simulink model "Copy_of_compare"  (R2018b)
settings: Solver=ode45  StartTime=0.0  StopTime=100  RelTol=1e-3
libraries: neural x108
(part 2 of 4)

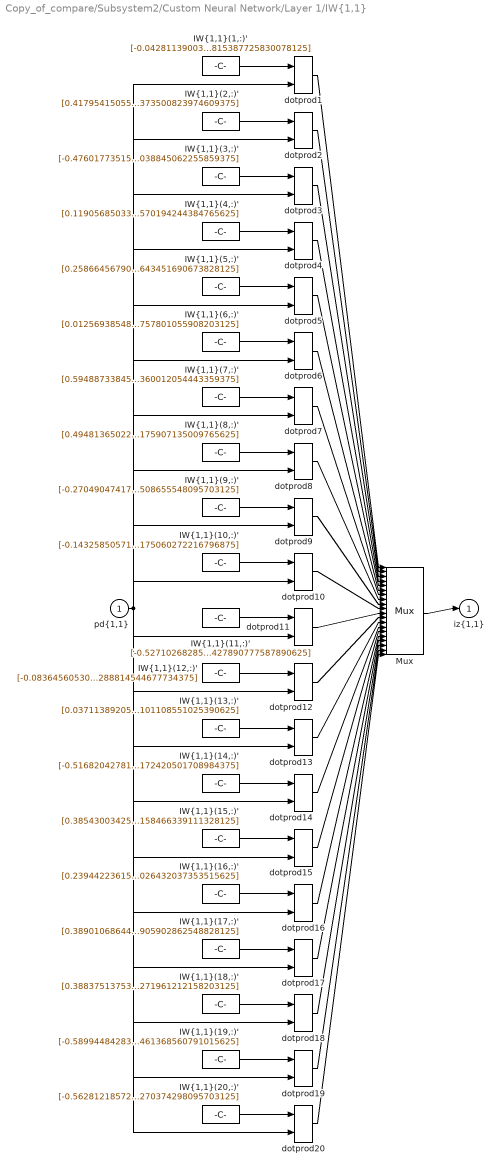
== system Copy_of_compare/Subsystem2/Custom Neural Network/Layer 1/IW{1,1} ==
  "pd{1,1}" : Inport  PortDimensions=4  SampleTime=1
      mask Display: e = 0.06;c1 = [120 230 180]/255;c2 = ([120 230 180]+0)/(256+128);c3 = ([120 230 180]+128)/(256+128);patch([0 1 1 0],[0 0 1 1],c1);patch([0 1 1 1-e 1-e 0+e],[0 0 1 1-e 0+e 0+e],c2);patch([0 0 1 1-e 0+e 0+e],[0 1 1 1-e 1-e 0+e],c3);plot([0 1 1 0 0],[0 0 1 1 0]);
  "IW{1,1}(1,:)'" : Constant  Value=[-0.042811390033023755119501174704055301845073699951171875;-0.34494124940580495053410459149745292961597442626953125;0.212181792987700124086813957546837627887725830078125;0.19703731840338456482442097694729454815387725830078125]
      mask Display: e = 0.06;c1 = [120 150 230]/255;c2 = ([120 150 230]+0)/383;c3 = ([120 150 230]+128)/383;patch([0 1 1 0],[0 0 1 1],c1);patch([0 1 1 1-e 1-e 0+e],[0 0 1 1-e 0+e 0+e],c2);patch([0 0 1 1-e 0+e 0+e],[0 1 1 1-e 1-e 0+e],c3);plot([0 1 1 0 0],[0 0 1 1 0]);disp('Weights');
  "IW{1,1}(10,:)'" : Constant  Value=[-0.1432585057147908458308194212804664857685565948486328125;-0.153266205858384185756193573979544453322887420654296875;0.49559029394590659034491864076699130237102508544921875;-0.07933482509106119795472267242075758986175060272216796875]
      mask Display: e = 0.06;c1 = [120 150 230]/255;c2 = ([120 150 230]+0)/383;c3 = ([120 150 230]+128)/383;patch([0 1 1 0],[0 0 1 1],c1);patch([0 1 1 1-e 1-e 0+e],[0 0 1 1-e 0+e 0+e],c2);patch([0 0 1 1-e 0+e 0+e],[0 1 1 1-e 1-e 0+e],c3);plot([0 1 1 0 0],[0 0 1 1 0]);disp('Weights');
  "IW{1,1}(11,:)'" : Constant  Value=[-0.5271026828588116774909622108680196106433868408203125;-0.19376380367271484050917251806822605431079864501953125;-0.50126266277864350850990149410790763795375823974609375;-0.1275131171211906500051469492973410524427890777587890625]
      mask Display: e = 0.06;c1 = [120 150 230]/255;c2 = ([120 150 230]+0)/383;c3 = ([120 150 230]+128)/383;patch([0 1 1 0],[0 0 1 1],c1);patch([0 1 1 1-e 1-e 0+e],[0 0 1 1-e 0+e 0+e],c2);patch([0 0 1 1-e 0+e 0+e],[0 1 1 1-e 1-e 0+e],c3);plot([0 1 1 0 0],[0 0 1 1 0]);disp('Weights');
  "IW{1,1}(12,:)'" : Constant  Value=[-0.083645605300920744529236117159598506987094879150390625;0.1272107414484172360769065335261984728276729583740234375;-0.1374343203091800968973501539949211291968822479248046875;0.66581955393483605032400873824371956288814544677734375]
      mask Display: e = 0.06;c1 = [120 150 230]/255;c2 = ([120 150 230]+0)/383;c3 = ([120 150 230]+128)/383;patch([0 1 1 0],[0 0 1 1],c1);patch([0 1 1 1-e 1-e 0+e],[0 0 1 1-e 0+e 0+e],c2);patch([0 0 1 1-e 0+e 0+e],[0 1 1 1-e 1-e 0+e],c3);plot([0 1 1 0 0],[0 0 1 1 0]);disp('Weights');
  "IW{1,1}(13,:)'" : Constant  Value=[0.03711389205480629394084957084487541578710079193115234375;-0.462899083442104508634429294033907353878021240234375;-0.2264716472284484527488501726111280731856822967529296875;0.4688615702267180385121037033968605101108551025390625]
      mask Display: e = 0.06;c1 = [120 150 230]/255;c2 = ([120 150 230]+0)/383;c3 = ([120 150 230]+128)/383;patch([0 1 1 0],[0 0 1 1],c1);patch([0 1 1 1-e 1-e 0+e],[0 0 1 1-e 0+e 0+e],c2);patch([0 0 1 1-e 0+e 0+e],[0 1 1 1-e 1-e 0+e],c3);plot([0 1 1 0 0],[0 0 1 1 0]);disp('Weights');
  "IW{1,1}(14,:)'" : Constant  Value=[-0.5168204278140742236047344704275019466876983642578125;0.45663111946031242904808777893777005374431610107421875;-0.51419835913847655728403651664848439395427703857421875;-0.09691171847871636602089751022504060529172420501708984375]
      mask Display: e = 0.06;c1 = [120 150 230]/255;c2 = ([120 150 230]+0)/383;c3 = ([120 150 230]+128)/383;patch([0 1 1 0],[0 0 1 1],c1);patch([0 1 1 1-e 1-e 0+e],[0 0 1 1-e 0+e 0+e],c2);patch([0 0 1 1-e 0+e 0+e],[0 1 1 1-e 1-e 0+e],c3);plot([0 1 1 0 0],[0 0 1 1 0]);disp('Weights');
  "IW{1,1}(15,:)'" : Constant  Value=[0.385430034255971387668893157751881517469882965087890625;-0.215305325209396214436452510199160315096378326416015625;-0.1868848258074100876502399160017375834286212921142578125;0.39665474045523041457528279352118261158466339111328125]
      mask Display: e = 0.06;c1 = [120 150 230]/255;c2 = ([120 150 230]+0)/383;c3 = ([120 150 230]+128)/383;patch([0 1 1 0],[0 0 1 1],c1);patch([0 1 1 1-e 1-e 0+e],[0 0 1 1-e 0+e 0+e],c2);patch([0 0 1 1-e 0+e 0+e],[0 1 1 1-e 1-e 0+e],c3);plot([0 1 1 0 0],[0 0 1 1 0]);disp('Weights');
  "IW{1,1}(16,:)'" : Constant  Value=[0.2394422361532615173285165610650437884032726287841796875;0.5573707637317522056719099055044353008270263671875;-0.44328627858535185612964824031223542988300323486328125;-0.20052230029704232183718204396427609026432037353515625]
      mask Display: e = 0.06;c1 = [120 150 230]/255;c2 = ([120 150 230]+0)/383;c3 = ([120 150 230]+128)/383;patch([0 1 1 0],[0 0 1 1],c1);patch([0 1 1 1-e 1-e 0+e],[0 0 1 1-e 0+e 0+e],c2);patch([0 0 1 1-e 0+e 0+e],[0 1 1 1-e 1-e 0+e],c3);plot([0 1 1 0 0],[0 0 1 1 0]);disp('Weights');
  "IW{1,1}(17,:)'" : Constant  Value=[0.38901068644869807311437170938006602227687835693359375;-0.427525166182410376602973656190442852675914764404296875;-0.443132878250084905058514550546533428132534027099609375;0.37252488448668785725459429158945567905902862548828125]
      mask Display: e = 0.06;c1 = [120 150 230]/255;c2 = ([120 150 230]+0)/383;c3 = ([120 150 230]+128)/383;patch([0 1 1 0],[0 0 1 1],c1);patch([0 1 1 1-e 1-e 0+e],[0 0 1 1-e 0+e 0+e],c2);patch([0 0 1 1-e 0+e 0+e],[0 1 1 1-e 1-e 0+e],c3);plot([0 1 1 0 0],[0 0 1 1 0]);disp('Weights');
  "IW{1,1}(18,:)'" : Constant  Value=[0.38837513753777053171489797023241408169269561767578125;-0.329414929396628364255406040683737955987453460693359375;0.447224063257221360334625614996184594929218292236328125;-0.293902664542561364857675698658567853271961212158203125]
      mask Display: e = 0.06;c1 = [120 150 230]/255;c2 = ([120 150 230]+0)/383;c3 = ([120 150 230]+128)/383;patch([0 1 1 0],[0 0 1 1],c1);patch([0 1 1 1-e 1-e 0+e],[0 0 1 1-e 0+e 0+e],c2);patch([0 0 1 1-e 0+e 0+e],[0 1 1 1-e 1-e 0+e],c3);plot([0 1 1 0 0],[0 0 1 1 0]);disp('Weights');
  "IW{1,1}(19,:)'" : Constant  Value=[-0.58994484283590320483625646375003270804882049560546875;-0.4543619457979339859576839444343931972980499267578125;-0.38699246687251276366481533841579221189022064208984375;-0.1299714765164118601692422316773445345461368560791015625]
      mask Display: e = 0.06;c1 = [120 150 230]/255;c2 = ([120 150 230]+0)/383;c3 = ([120 150 230]+128)/383;patch([0 1 1 0],[0 0 1 1],c1);patch([0 1 1 1-e 1-e 0+e],[0 0 1 1-e 0+e 0+e],c2);patch([0 0 1 1-e 0+e 0+e],[0 1 1 1-e 1-e 0+e],c3);plot([0 1 1 0 0],[0 0 1 1 0]);disp('Weights');
  "IW{1,1}(2,:)'" : Constant  Value=[0.417954150552907910398658941630856133997440338134765625;0.37950717584964566153615805887966416776180267333984375;-0.444355699691141747820211094222031533718109130859375;0.40455774770315766630801590508781373500823974609375]
      mask Display: e = 0.06;c1 = [120 150 230]/255;c2 = ([120 150 230]+0)/383;c3 = ([120 150 230]+128)/383;patch([0 1 1 0],[0 0 1 1],c1);patch([0 1 1 1-e 1-e 0+e],[0 0 1 1-e 0+e 0+e],c2);patch([0 0 1 1-e 0+e 0+e],[0 1 1 1-e 1-e 0+e],c3);plot([0 1 1 0 0],[0 0 1 1 0]);disp('Weights');
  "IW{1,1}(20,:)'" : Constant  Value=[-0.56281218572056845861339979819604195654392242431640625;-0.1531865678348197923330786807127879001200199127197265625;0.32894636374948527102191064841463230550289154052734375;-0.11506127596662703294061458336727810092270374298095703125]
      mask Display: e = 0.06;c1 = [120 150 230]/255;c2 = ([120 150 230]+0)/383;c3 = ([120 150 230]+128)/383;patch([0 1 1 0],[0 0 1 1],c1);patch([0 1 1 1-e 1-e 0+e],[0 0 1 1-e 0+e 0+e],c2);patch([0 0 1 1-e 0+e 0+e],[0 1 1 1-e 1-e 0+e],c3);plot([0 1 1 0 0],[0 0 1 1 0]);disp('Weights');
  "IW{1,1}(3,:)'" : Constant  Value=[-0.476017735150680909583797983941622078418731689453125;0.372659870345571853089694513982976786792278289794921875;0.15761264234491967339835127859259955585002899169921875;-0.301498932852593437559107769629918038845062255859375]
      mask Display: e = 0.06;c1 = [120 150 230]/255;c2 = ([120 150 230]+0)/383;c3 = ([120 150 230]+128)/383;patch([0 1 1 0],[0 0 1 1],c1);patch([0 1 1 1-e 1-e 0+e],[0 0 1 1-e 0+e 0+e],c2);patch([0 0 1 1-e 0+e 0+e],[0 1 1 1-e 1-e 0+e],c3);plot([0 1 1 0 0],[0 0 1 1 0]);disp('Weights');
  "IW{1,1}(4,:)'" : Constant  Value=[0.1190568503323596039056297968272701837122440338134765625;0.025251810519317963166230356364394538104534149169921875;-0.01463313633015732827258315040808156481944024562835693359375;0.0799177967721290960501079325695172883570194244384765625]
      mask Display: e = 0.06;c1 = [120 150 230]/255;c2 = ([120 150 230]+0)/383;c3 = ([120 150 230]+128)/383;patch([0 1 1 0],[0 0 1 1],c1);patch([0 1 1 1-e 1-e 0+e],[0 0 1 1-e 0+e 0+e],c2);patch([0 0 1 1-e 0+e 0+e],[0 1 1 1-e 1-e 0+e],c3);plot([0 1 1 0 0],[0 0 1 1 0]);disp('Weights');
  "IW{1,1}(5,:)'" : Constant  Value=[0.2586645679057075764006867757416330277919769287109375;-0.359798037926290892318803571470198221504688262939453125;0.49791321437721602904957762802951037883758544921875;-0.2408924072199911947667061440370162017643451690673828125]
      mask Display: e = 0.06;c1 = [120 150 230]/255;c2 = ([120 150 230]+0)/383;c3 = ([120 150 230]+128)/383;patch([0 1 1 0],[0 0 1 1],c1);patch([0 1 1 1-e 1-e 0+e],[0 0 1 1-e 0+e 0+e],c2);patch([0 0 1 1-e 0+e 0+e],[0 1 1 1-e 1-e 0+e],c3);plot([0 1 1 0 0],[0 0 1 1 0]);disp('Weights');
  "IW{1,1}(6,:)'" : Constant  Value=[0.01256938548635226811367449073486568522639572620391845703125;0.422855987628569407466017082697362639009952545166015625;0.482605939133784911376778836711309850215911865234375;-0.478909325852367839804202276354772038757801055908203125]
      mask Display: e = 0.06;c1 = [120 150 230]/255;c2 = ([120 150 230]+0)/383;c3 = ([120 150 230]+128)/383;patch([0 1 1 0],[0 0 1 1],c1);patch([0 1 1 1-e 1-e 0+e],[0 0 1 1-e 0+e 0+e],c2);patch([0 0 1 1-e 0+e 0+e],[0 1 1 1-e 1-e 0+e],c3);plot([0 1 1 0 0],[0 0 1 1 0]);disp('Weights');
  "IW{1,1}(7,:)'" : Constant  Value=[0.5948873384524977492304742554551921784877777099609375;0.281306962804711513381761278651538304984569549560546875;-0.1572109737119190830956227955539361573755741119384765625;0.1660798915358044636203516120076528750360012054443359375]
      mask Display: e = 0.06;c1 = [120 150 230]/255;c2 = ([120 150 230]+0)/383;c3 = ([120 150 230]+128)/383;patch([0 1 1 0],[0 0 1 1],c1);patch([0 1 1 1-e 1-e 0+e],[0 0 1 1-e 0+e 0+e],c2);patch([0 0 1 1-e 0+e 0+e],[0 1 1 1-e 1-e 0+e],c3);plot([0 1 1 0 0],[0 0 1 1 0]);disp('Weights');
  "IW{1,1}(8,:)'" : Constant  Value=[0.494813650227310108942191391179221682250499725341796875;-0.1661270735577930202087060251869843341410160064697265625;-0.323120860559985623172707391859148629009723663330078125;-0.120857806854206606406165747102932073175907135009765625]
      mask Display: e = 0.06;c1 = [120 150 230]/255;c2 = ([120 150 230]+0)/383;c3 = ([120 150 230]+128)/383;patch([0 1 1 0],[0 0 1 1],c1);patch([0 1 1 1-e 1-e 0+e],[0 0 1 1-e 0+e 0+e],c2);patch([0 0 1 1-e 0+e 0+e],[0 1 1 1-e 1-e 0+e],c3);plot([0 1 1 0 0],[0 0 1 1 0]);disp('Weights');
  "IW{1,1}(9,:)'" : Constant  Value=[-0.27049047417204652443700751973665319383144378662109375;-0.030493674231205934732624740490791737101972103118896484375;-0.30275890613240985516085856943391263484954833984375;0.32392632672577914565437140481662936508655548095703125]
      mask Display: e = 0.06;c1 = [120 150 230]/255;c2 = ([120 150 230]+0)/383;c3 = ([120 150 230]+128)/383;patch([0 1 1 0],[0 0 1 1],c1);patch([0 1 1 1-e 1-e 0+e],[0 0 1 1-e 0+e 0+e],c2);patch([0 0 1 1-e 0+e 0+e],[0 1 1 1-e 1-e 0+e],c3);plot([0 1 1 0 0],[0 0 1 1 0]);disp('Weights');
  Mux : Mux  Inputs=20
      mask Display: e = 0.06;c1 = [120 150 230]/255;c2 = ([120 150 230]+0)/383;c3 = ([120 150 230]+128)/383;patch([0 1 1 0],[0 0 1 1],c1);patch([0 1 1 1-e 1-e 0+e],[0 0 1 1-e 0+e 0+e],c2);patch([0 0 1 1-e 0+e 0+e],[0 1 1 1-e 1-e 0+e],c3);plot([0 1 1 0 0],[0 0 1 1 0]);disp('Mux');
  dotprod{1..20} (20 alike) : neural/Weight Functions/dotprod
  "iz{1,1}" : Outport
      mask Display: e = 0.06;c1 = [120 230 180]/255;c2 = ([120 230 180]+0)/(256+128);c3 = ([120 230 180]+128)/(256+128);patch([0 1 1 0],[0 0 1 1],c1);patch([0 1 1 1-e 1-e 0+e],[0 0 1 1-e 0+e 0+e],c2);patch([0 0 1 1-e 0+e 0+e],[0 1 1 1-e 1-e 0+e],c3);plot([0 1 1 0 0],[0 0 1 1 0]);
  wires:
  "IW{1,1}(1,:)'"/1 -> dotprod1/1
  "pd{1,1}"/1 -> dotprod1/2, dotprod2/2, dotprod3/2, dotprod4/2, dotprod5/2, dotprod6/2, dotprod7/2, dotprod8/2, dotprod9/2, dotprod10/2, dotprod11/2, dotprod12/2, dotprod13/2, dotprod14/2, dotprod15/2, dotprod16/2, dotprod17/2, dotprod18/2, dotprod19/2, dotprod20/2
  dotprod1/1 -> Mux/1
  "IW{1,1}(2,:)'"/1 -> dotprod2/1
  dotprod2/1 -> Mux/2
  "IW{1,1}(3,:)'"/1 -> dotprod3/1
  dotprod3/1 -> Mux/3
  "IW{1,1}(4,:)'"/1 -> dotprod4/1
  dotprod4/1 -> Mux/4
  "IW{1,1}(5,:)'"/1 -> dotprod5/1
  dotprod5/1 -> Mux/5
  "IW{1,1}(6,:)'"/1 -> dotprod6/1
  dotprod6/1 -> Mux/6
  "IW{1,1}(7,:)'"/1 -> dotprod7/1
  dotprod7/1 -> Mux/7
  "IW{1,1}(8,:)'"/1 -> dotprod8/1
  dotprod8/1 -> Mux/8
  "IW{1,1}(9,:)'"/1 -> dotprod9/1
  dotprod9/1 -> Mux/9
  "IW{1,1}(10,:)'"/1 -> dotprod10/1
  dotprod10/1 -> Mux/10
  "IW{1,1}(11,:)'"/1 -> dotprod11/1
  dotprod11/1 -> Mux/11
  "IW{1,1}(12,:)'"/1 -> dotprod12/1
  dotprod12/1 -> Mux/12
  "IW{1,1}(13,:)'"/1 -> dotprod13/1
  dotprod13/1 -> Mux/13
  "IW{1,1}(14,:)'"/1 -> dotprod14/1
  dotprod14/1 -> Mux/14
  "IW{1,1}(15,:)'"/1 -> dotprod15/1
  dotprod15/1 -> Mux/15
  "IW{1,1}(16,:)'"/1 -> dotprod16/1
  dotprod16/1 -> Mux/16
  "IW{1,1}(17,:)'"/1 -> dotprod17/1
  dotprod17/1 -> Mux/17
  "IW{1,1}(18,:)'"/1 -> dotprod18/1
  dotprod18/1 -> Mux/18
  "IW{1,1}(19,:)'"/1 -> dotprod19/1
  dotprod19/1 -> Mux/19
  "IW{1,1}(20,:)'"/1 -> dotprod20/1
  dotprod20/1 -> Mux/20
  Mux/1 -> "iz{1,1}"/1

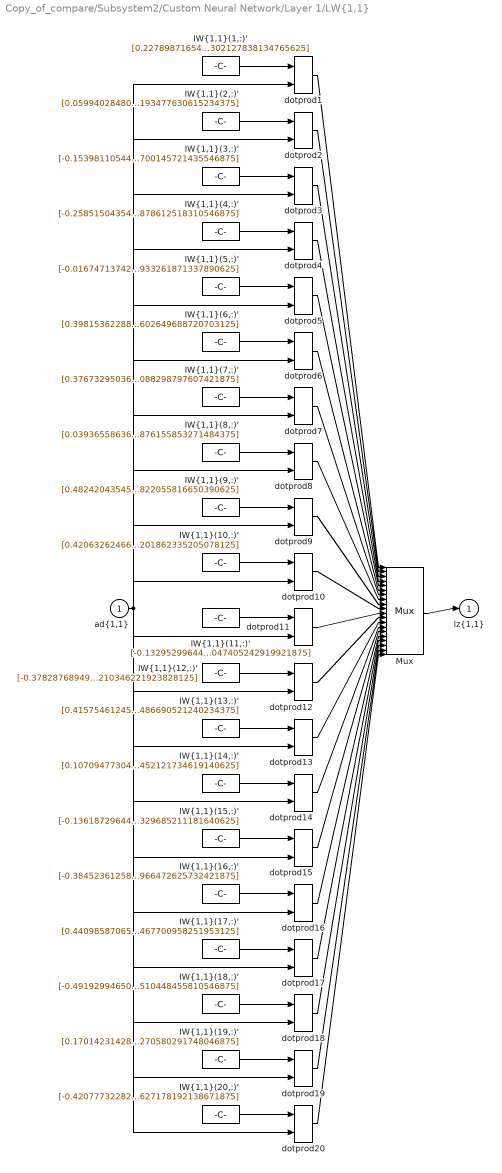
== system Copy_of_compare/Subsystem2/Custom Neural Network/Layer 1/LW{1,1} ==
  "ad{1,1}" : Inport  PortDimensions=20  SampleTime=1
      mask Display: e = 0.06;c1 = [120 230 180]/255;c2 = ([120 230 180]+0)/(256+128);c3 = ([120 230 180]+128)/(256+128);patch([0 1 1 0],[0 0 1 1],c1);patch([0 1 1 1-e 1-e 0+e],[0 0 1 1-e 0+e 0+e],c2);patch([0 0 1 1-e 0+e 0+e],[0 1 1 1-e 1-e 0+e],c3);plot([0 1 1 0 0],[0 0 1 1 0]);
  "IW{1,1}(1,:)'" : Constant  Value=[0.2278987165494096578388649732005433179438114166259765625;0.240540154904058389728760403158958069980144500732421875;-0.08228071789715719897007062400007271207869052886962890625;0.4457988335202587304451071759103797376155853271484375;-0.23129699864569508438449929599300958216190338134765625;-0.49692828504273933720725153762032277882099151611328125;0.38560473208843759618247304388205520808696746826171875;0.31956777070472852653182371795992366969585418701171875;0.1656064949527651652960713590800878591835498809814453125;0.229070693094035660042351310039521194994449615478515625;-0.475851979993766105447861036736867390573024749755859375;0.31630195271679417690080526881502009928226470947265625;0.49015943893010571752455462046782486140727996826171875;-0.50065157873258236964630896181915886700153350830078125;-0.45776780495111413227249386181938461959362030029296875;0.2098533389682639693774035549722611904144287109375;0.38657180100997201588342022660071961581707000732421875;0.240641344614608454488546840366325341165065765380859375;-0.30911232252311748869288976493407972157001495361328125;0.07903324281619496238793232123498455621302127838134765625]
      mask Display: e = 0.06;c1 = [120 150 230]/255;c2 = ([120 150 230]+0)/383;c3 = ([120 150 230]+128)/383;patch([0 1 1 0],[0 0 1 1],c1);patch([0 1 1 1-e 1-e 0+e],[0 0 1 1-e 0+e 0+e],c2);patch([0 0 1 1-e 0+e 0+e],[0 1 1 1-e 1-e 0+e],c3);plot([0 1 1 0 0],[0 0 1 1 0]);disp('weights');
  "IW{1,1}(10,:)'" : Constant  Value=[0.420632624664030119188140588448732160031795501708984375;0.429185444508361990667566487900330685079097747802734375;-0.491659080709817175591780369359184987843036651611328125;0.182452654614607079341936923810862936079502105712890625;-0.10699046596342180748262506995160947553813457489013671875;0.1602960437006126503955982798288459889590740203857421875;-0.38946695359310312678502441485761664807796478271484375;-0.23785342454607505402464084909297525882720947265625;0.09697167013946524083412015215799328871071338653564453125;-0.2307044267848055996150691271395771764218807220458984375;0.27990512871394057636820207335404120385646820068359375;0.3074695770440818431978868829901330173015594482421875;-0.49869450365044720729912341994349844753742218017578125;0.212638380584271258211259691961458884179592132568359375;0.0196244391094952570775422628912565414793789386749267578125;-0.155944109151455012618470163943129591643810272216796875;0.469563664574393968553778222485561855137348175048828125;0.271650147852854517704912495901226066052913665771484375;0.514697400127334336872308995225466787815093994140625;-0.463282954366107724286649727218900807201862335205078125]
      mask Display: e = 0.06;c1 = [120 150 230]/255;c2 = ([120 150 230]+0)/383;c3 = ([120 150 230]+128)/383;patch([0 1 1 0],[0 0 1 1],c1);patch([0 1 1 1-e 1-e 0+e],[0 0 1 1-e 0+e 0+e],c2);patch([0 0 1 1-e 0+e 0+e],[0 1 1 1-e 1-e 0+e],c3);plot([0 1 1 0 0],[0 0 1 1 0]);disp('weights');
  "IW{1,1}(11,:)'" : Constant  Value=[-0.13295299644515246040299416563357226550579071044921875;-0.34257970274611437844214378856122493743896484375;-0.50546742207309069971898907169816084206104278564453125;0.375317987307353051473768346113502047955989837646484375;0.293111656529973618745543717523105442523956298828125;-0.4780711225226854654835051405825652182102203369140625;-0.29780200740318452101718094127136282622814178466796875;0.12431875943552746222042770796178956516087055206298828125;0.1488731855108570700796377650476642884314060211181640625;0.47588212639451510366228603743365965783596038818359375;-0.2544601172016609513804041853290982544422149658203125;-0.387733186112341365880951116196229122579097747802734375;-0.178865737611743902402139383411849848926067352294921875;-0.36554438569003178116645358386449515819549560546875;0.265494376935527187644225932672270573675632476806640625;-0.145739478578150116749867493126657791435718536376953125;-0.1630710952019509552002318741870112717151641845703125;-0.420982141038813761912962263522786088287830352783203125;-0.318278423537587451530583848580135963857173919677734375;-0.08046330758533119797970556419386412017047405242919921875]
      mask Display: e = 0.06;c1 = [120 150 230]/255;c2 = ([120 150 230]+0)/383;c3 = ([120 150 230]+128)/383;patch([0 1 1 0],[0 0 1 1],c1);patch([0 1 1 1-e 1-e 0+e],[0 0 1 1-e 0+e 0+e],c2);patch([0 0 1 1-e 0+e 0+e],[0 1 1 1-e 1-e 0+e],c3);plot([0 1 1 0 0],[0 0 1 1 0]);disp('weights');
  "IW{1,1}(12,:)'" : Constant  Value=[-0.378287689491962009213921191985718905925750732421875;0.31412463184470540422665862934081815183162689208984375;-0.245211026062742920572645743959583342075347900390625;-0.347387547677588059968911693431437015533447265625;-0.5031677654191166748631758309784345328807830810546875;-0.50758261729631259928652298185625113546848297119140625;0.37116161778317968700235951473587192595005035400390625;-0.03775716422149082152071031259765732102096080780029296875;-0.04605910262436473112668267049230053089559078216552734375;0.0104202638426654503600587986511527560651302337646484375;0.1388820306765665979487067716036108322441577911376953125;0.32356457862817589177240051867556758224964141845703125;0.00903262123542868111680803622220992110669612884521484375;0.545086378847996488872240661294199526309967041015625;0.054844572033606098226954372876207344233989715576171875;-0.12227603828467183133543727535652578808367252349853515625;0.52393929318664655969683963121497072279453277587890625;-0.1110905758660236941626209272726555354893207550048828125;0.54684918251084091433966705153579823672771453857421875;-0.241502604628337724790299034793861210346221923828125]
      mask Display: e = 0.06;c1 = [120 150 230]/255;c2 = ([120 150 230]+0)/383;c3 = ([120 150 230]+128)/383;patch([0 1 1 0],[0 0 1 1],c1);patch([0 1 1 1-e 1-e 0+e],[0 0 1 1-e 0+e 0+e],c2);patch([0 0 1 1-e 0+e 0+e],[0 1 1 1-e 1-e 0+e],c3);plot([0 1 1 0 0],[0 0 1 1 0]);disp('weights');
  "IW{1,1}(13,:)'" : Constant  Value=[0.41575461245577349789215304554090835154056549072265625;-0.409758839927184037588148157738032750785350799560546875;0.0292141310860018731110354650581939495168626308441162109375;0.32632919895820433620059475288144312798976898193359375;-0.39978185631407348044064065106795169413089752197265625;-0.419945798962307659252246594405733048915863037109375;-0.1446788768866233698684453656824189238250255584716796875;-0.33483109447959369386893513365066610276699066162109375;-0.039567165528868041002308331144377007149159908294677734375;0.29233486785391515905274673059466294944286346435546875;-0.322702359571785724057235711370594799518585205078125;0.346982308737791067532185707023018039762973785400390625;-0.00956612543968184993181669284467716352082788944244384765625;-0.3877596423322573482295183566748164594173431396484375;-0.35300446726813017317425646979245357215404510498046875;0.2962997531462061573392929858528077602386474609375;-0.40146500486877789715123299174592830240726470947265625;-0.377307450578544034680561480854521505534648895263671875;0.407805095951260521136561010280274786055088043212890625;-0.1819632532644864519877359043675824068486690521240234375]
      mask Display: e = 0.06;c1 = [120 150 230]/255;c2 = ([120 150 230]+0)/383;c3 = ([120 150 230]+128)/383;patch([0 1 1 0],[0 0 1 1],c1);patch([0 1 1 1-e 1-e 0+e],[0 0 1 1-e 0+e 0+e],c2);patch([0 0 1 1-e 0+e 0+e],[0 1 1 1-e 1-e 0+e],c3);plot([0 1 1 0 0],[0 0 1 1 0]);disp('weights');
  "IW{1,1}(14,:)'" : Constant  Value=[0.1070947730439226475152025841452996246516704559326171875;-0.271684022564260552190518183124368079006671905517578125;0.28236026004421599377991469737025909125804901123046875;0.2240856228544926553869487406700500287115573883056640625;-0.424180068223444506347874494167626835405826568603515625;0.09805112035332404218923585403899778611958026885986328125;-0.257571951610501781448903102500480599701404571533203125;-0.0929025916780819860374407426206744275987148284912109375;0.463081155692898149833780507833580486476421356201171875;0.32611395715227597946750393020920455455780029296875;-0.27906063380379120264507264437270350754261016845703125;-0.461085781794401849964515349711291491985321044921875;0.077706195310071723980627211858518421649932861328125;-0.30058122236647388803021385683678090572357177734375;0.4548280591144233664380180925945751368999481201171875;0.1008924803782029477883241952440585009753704071044921875;-0.375142648760853791856106909108348190784454345703125;-0.41173315079330163879234305568388663232326507568359375;-0.262394554640659916078249125348520465195178985595703125;-0.056615575605880132104008595206323661841452121734619140625]
      mask Display: e = 0.06;c1 = [120 150 230]/255;c2 = ([120 150 230]+0)/383;c3 = ([120 150 230]+128)/383;patch([0 1 1 0],[0 0 1 1],c1);patch([0 1 1 1-e 1-e 0+e],[0 0 1 1-e 0+e 0+e],c2);patch([0 0 1 1-e 0+e 0+e],[0 1 1 1-e 1-e 0+e],c3);plot([0 1 1 0 0],[0 0 1 1 0]);disp('weights');
  "IW{1,1}(15,:)'" : Constant  Value=[-0.136187296441313610007028955806163139641284942626953125;0.209037331339636534011106050456874072551727294921875;-0.32626772882534027520051722603966481983661651611328125;-0.462079150500124213873931466878275386989116668701171875;-0.285236058869271780213949796234373934566974639892578125;0.1559960849596407073125448050632257945835590362548828125;0.36825294505482997209355744416825473308563232421875;0.18261079235679178456308591194101609289646148681640625;0.0492753080605025928218054787066648714244365692138671875;0.138081756097673480354615094256587326526641845703125;0.07186485845076993894675609908517799340188503265380859375;-0.4007107673316190332712949384585954248905181884765625;0.430359673196610781342741347543778829276561737060546875;0.4609101603710115124812318754266016185283660888671875;-0.404191060521045975040266284850076772272586822509765625;-0.334065431476544050237720284712850116193294525146484375;-0.447605082750429150717508264278876595199108123779296875;-0.424280447044566688674649412860162556171417236328125;-0.372089526528038394559416701667942106723785400390625;-0.1983326147027272556844224027372547425329685211181640625]
      mask Display: e = 0.06;c1 = [120 150 230]/255;c2 = ([120 150 230]+0)/383;c3 = ([120 150 230]+128)/383;patch([0 1 1 0],[0 0 1 1],c1);patch([0 1 1 1-e 1-e 0+e],[0 0 1 1-e 0+e 0+e],c2);patch([0 0 1 1-e 0+e 0+e],[0 1 1 1-e 1-e 0+e],c3);plot([0 1 1 0 0],[0 0 1 1 0]);disp('weights');
  "IW{1,1}(16,:)'" : Constant  Value=[-0.384523612583706597689570116926915943622589111328125;-0.206157590542222102225622393234516493976116180419921875;0.4554611951382001588939374414621852338314056396484375;0.49174573636799523423945856848149560391902923583984375;-0.1801231476021115385233173356027691625058650970458984375;0.4683739136963203097963059917674399912357330322265625;0.394822850463422636568822099434328265488147735595703125;0.391845140376515799207624013433814980089664459228515625;0.06459290894014728390271073976691695861518383026123046875;-0.34207481769281422590012198270414955914020538330078125;-0.490312179861580654804953383063548244535923004150390625;-0.045903438096631769826938551659623044542968273162841796875;0.439061671021340360621110221472918055951595306396484375;0.10461216405642752291793584618062595836818218231201171875;0.2258046443601937625089703942649066448211669921875;-0.416842953303650565199944821870303712785243988037109375;0.18497573731176597533476524404250085353851318359375;0.06843741391665482398654063445064821280539035797119140625;-0.108158723682227952966883322005742229521274566650390625;0.19655617248948764608229566874797455966472625732421875]
      mask Display: e = 0.06;c1 = [120 150 230]/255;c2 = ([120 150 230]+0)/383;c3 = ([120 150 230]+128)/383;patch([0 1 1 0],[0 0 1 1],c1);patch([0 1 1 1-e 1-e 0+e],[0 0 1 1-e 0+e 0+e],c2);patch([0 0 1 1-e 0+e 0+e],[0 1 1 1-e 1-e 0+e],c3);plot([0 1 1 0 0],[0 0 1 1 0]);disp('weights');
  "IW{1,1}(17,:)'" : Constant  Value=[0.44098587065739192070168428472243249416351318359375;-0.08788059273859938347328579766326583921909332275390625;-0.308675876398948501044827708028606139123439788818359375;-0.221486569567091506893774521813611499965190887451171875;0.2178678865951073628792755698668770492076873779296875;-0.289200773370994423938640238702646456658840179443359375;0.35306632808482019125762008115998469293117523193359375;-0.444884415917694620024036566974245943129062652587890625;-0.199324943462346693134890074361464940011501312255859375;-0.08840657649147143359869005507789552211761474609375;-0.4380941991671647439687831138144247233867645263671875;0.01346592043859511089731739730268600396811962127685546875;-0.47008827633134420143079523768392391502857208251953125;-0.20000214664542592668539100486668758094310760498046875;0.2742024362016126648455838221707381308078765869140625;-0.37841706486119919272681499933241866528987884521484375;0.01755574999820135040362600875596399419009685516357421875;-0.335116990061384678600830966388457454741001129150390625;0.16408210758615771052149057140923105180263519287109375;0.44147467938079476557078351106611080467700958251953125]
      mask Display: e = 0.06;c1 = [120 150 230]/255;c2 = ([120 150 230]+0)/383;c3 = ([120 150 230]+128)/383;patch([0 1 1 0],[0 0 1 1],c1);patch([0 1 1 1-e 1-e 0+e],[0 0 1 1-e 0+e 0+e],c2);patch([0 0 1 1-e 0+e 0+e],[0 1 1 1-e 1-e 0+e],c3);plot([0 1 1 0 0],[0 0 1 1 0]);disp('weights');
  "IW{1,1}(18,:)'" : Constant  Value=[-0.491929946506200088673921300141955725848674774169921875;-0.2126767242213216391188979059734265320003032684326171875;-0.1009912537251317077302559255258529447019100189208984375;0.3217560834001089720146637773723341524600982666015625;0.051956008299841281716791030476088053546845912933349609375;-0.1660321893331526965642552795543451793491840362548828125;0.0272606663276684334229482686851042672060430049896240234375;0.491487382911402981289228364403243176639080047607421875;-0.354138503368337353993666738460888154804706573486328125;0.2047296393810319747874615359251038171350955963134765625;0.423050942762800030738645773453754372894763946533203125;0.370056287706793940461835745736607350409030914306640625;0.04510904995247948245928881760846707038581371307373046875;-0.403977073562105160053903318839729763567447662353515625;0.238067026591629649079351338514243252575397491455078125;0.460926551166004505599715912467218004167079925537109375;0.307803449094200265445664399521774612367153167724609375;-0.444383412258365917413271972691291011869907379150390625;-0.1183301293074575932795511334916227497160434722900390625;0.223305523038261621859845718063297681510448455810546875]
      mask Display: e = 0.06;c1 = [120 150 230]/255;c2 = ([120 150 230]+0)/383;c3 = ([120 150 230]+128)/383;patch([0 1 1 0],[0 0 1 1],c1);patch([0 1 1 1-e 1-e 0+e],[0 0 1 1-e 0+e 0+e],c2);patch([0 0 1 1-e 0+e 0+e],[0 1 1 1-e 1-e 0+e],c3);plot([0 1 1 0 0],[0 0 1 1 0]);disp('weights');
  "IW{1,1}(19,:)'" : Constant  Value=[0.1701423142892309059437394580527325160801410675048828125;-0.411160005228003611055243027294636704027652740478515625;0.04775542972130684959974900039014755748212337493896484375;0.2284830513994409451061784466219251044094562530517578125;-0.07416597601648027004994645494662108831107616424560546875;0.058993659299435431686564612618894898332655429840087890625;-0.043994833927363745373906311897371779195964336395263671875;0.5347552742001904224622421679669059813022613525390625;-0.205233087407502790000535242143087089061737060546875;-0.06123054241270009523390172034851275384426116943359375;0.2382264629099061503669787498438381589949131011962890625;-0.2471133906297690863151927942453767172992229461669921875;-0.354185081063232154452435906932805664837360382080078125;-0.56028937632563480253367060868185944855213165283203125;0.242926896839649353321277658324106596410274505615234375;-0.202115344162328958166341408286825753748416900634765625;0.55654225518627431501528235457953996956348419189453125;-0.1141277041438499839642872757394798099994659423828125;0.298276236068890365782380058590206317603588104248046875;-0.42325436819033679380908097300562076270580291748046875]
      mask Display: e = 0.06;c1 = [120 150 230]/255;c2 = ([120 150 230]+0)/383;c3 = ([120 150 230]+128)/383;patch([0 1 1 0],[0 0 1 1],c1);patch([0 1 1 1-e 1-e 0+e],[0 0 1 1-e 0+e 0+e],c2);patch([0 0 1 1-e 0+e 0+e],[0 1 1 1-e 1-e 0+e],c3);plot([0 1 1 0 0],[0 0 1 1 0]);disp('weights');
  "IW{1,1}(2,:)'" : Constant  Value=[0.05994028480322521890144571443670429289340972900390625;-0.08139306170899605896718043140936060808598995208740234375;0.37859367841592528325378452791483141481876373291015625;-0.28921655327229156551283040244015865027904510498046875;-0.392439976848181715229912924769450910389423370361328125;0.396248727965390068472828488665982149541378021240234375;-0.3554873052677731681825434861821122467517852783203125;-0.2112195004145205612378077830726397223770618438720703125;0.08326096933293403168363511213101446628570556640625;0.37248571015998155342430209202575497329235076904296875;0.43360619759672258677341005750349722802639007568359375;0.282109436908400679211439410210005007684230804443359375;0.3373217412508566770412699042935855686664581298828125;0.1598161592246870321698537509291782043874263763427734375;0.451645495361196636086020816946984268724918365478515625;0.225318140185007786957527287086122669279575347900390625;-0.07006372872089793035765836748396395705640316009521484375;-0.429360930531992146530484433242236264050006866455078125;-0.299745954789107871274467242983519099652767181396484375;-0.1760596854637484776073819148223265074193477630615234375]
      mask Display: e = 0.06;c1 = [120 150 230]/255;c2 = ([120 150 230]+0)/383;c3 = ([120 150 230]+128)/383;patch([0 1 1 0],[0 0 1 1],c1);patch([0 1 1 1-e 1-e 0+e],[0 0 1 1-e 0+e 0+e],c2);patch([0 0 1 1-e 0+e 0+e],[0 1 1 1-e 1-e 0+e],c3);plot([0 1 1 0 0],[0 0 1 1 0]);disp('weights');
  "IW{1,1}(20,:)'" : Constant  Value=[-0.4207773228277627008964145716163329780101776123046875;0.61274610734971990400055119607714004814624786376953125;-0.46890358589581782045030422523268498480319976806640625;0.421025844859461317870596985812881030142307281494140625;-0.254298671278955612518046791592496447265148162841796875;0.253825658806738962969262729529873467981815338134765625;0.06416183898043288647006221481206011958420276641845703125;0.276316001132758282121670845299377106130123138427734375;0.1493101435030437518225454596176859922707080841064453125;-0.338446172666960920505374588174163363873958587646484375;-0.1197449463928856594474581243048305623233318328857421875;0.333161081431593952828507099184207618236541748046875;-0.01897741486999000859459130197137710638344287872314453125;0.1261536684585937428959567796482588164508342742919921875;0.67982698446328726493703697997261770069599151611328125;0.0749081099411582906899553790935897268354892730712890625;0.374586859509620229147230929811485111713409423828125;-0.03891781703874953868282915436793700791895389556884765625;-0.087120705006512089152437283701146952807903289794921875;-0.036398370094171510202851749227193067781627178192138671875]
      mask Display: e = 0.06;c1 = [120 150 230]/255;c2 = ([120 150 230]+0)/383;c3 = ([120 150 230]+128)/383;patch([0 1 1 0],[0 0 1 1],c1);patch([0 1 1 1-e 1-e 0+e],[0 0 1 1-e 0+e 0+e],c2);patch([0 0 1 1-e 0+e 0+e],[0 1 1 1-e 1-e 0+e],c3);plot([0 1 1 0 0],[0 0 1 1 0]);disp('weights');
  "IW{1,1}(3,:)'" : Constant  Value=[-0.1539811054447259019983818006949150003492832183837890625;-0.2274987476907101846546055412545683793723583221435546875;0.286517531317783291644474275017273612320423126220703125;-9.4276511529738939686173804233249029493890702724456787109375e-05;-0.49053060353080557565164099287358112633228302001953125;-0.313030491451828873916696238666190765798091888427734375;-0.3658368261830309275950412484235130250453948974609375;-0.378278173927990624125783369890996254980564117431640625;0.50047347942805886500394763061194680631160736083984375;-0.1983560574684938015987967219189158640801906585693359375;0.2344843868306323575456673324879375286400318145751953125;0.362707499239886821396083860236103646457195281982421875;0.2053939939299573025355272193337441422045230865478515625;-0.466207691386206046768592159423860721290111541748046875;0.21395563541551887443148416423355229198932647705078125;-0.4059408516154994206459605265990830957889556884765625;0.09096149913632174677236008619729545898735523223876953125;0.47838015297459091090814808922004885971546173095703125;0.280847689582235882088667722200625576078891754150390625;0.03654710138079979298009192234530928544700145721435546875]
      mask Display: e = 0.06;c1 = [120 150 230]/255;c2 = ([120 150 230]+0)/383;c3 = ([120 150 230]+128)/383;patch([0 1 1 0],[0 0 1 1],c1);patch([0 1 1 1-e 1-e 0+e],[0 0 1 1-e 0+e 0+e],c2);patch([0 0 1 1-e 0+e 0+e],[0 1 1 1-e 1-e 0+e],c3);plot([0 1 1 0 0],[0 0 1 1 0]);disp('weights');
  "IW{1,1}(4,:)'" : Constant  Value=[-0.258515043540460565107963475384167395532131195068359375;-0.4211939696771513919060225816792808473110198974609375;0.52216714859414603555620715269469656050205230712890625;-0.393692104389318731083591274000355042517185211181640625;-0.369465419709244347057364166175830177962779998779296875;0.2025300288650582480887152314608101733028888702392578125;-0.51664031300845947303201910472125746309757232666015625;0.318875824416838538066798491854569874703884124755859375;0.40125045776646672823773087657173164188861846923828125;0.50617791462088879139713526456034742295742034912109375;0.37477002720246577194274095745640806853771209716796875;0.308205903710022710573213089446653611958026885986328125;-0.3368272811142547507046174359857104718685150146484375;-0.395270413802351061605122595210559666156768798828125;-0.260207488946448239897080156879383139312267303466796875;0.1890510736151615189815089479452581144869327545166015625;0.2207311215862742537208163184914155863225460052490234375;0.11392669327151348779292305835042498074471950531005859375;0.13204164178805399831873046423424966633319854736328125;0.40005168727957407526218958082608878612518310546875]
      mask Display: e = 0.06;c1 = [120 150 230]/255;c2 = ([120 150 230]+0)/383;c3 = ([120 150 230]+128)/383;patch([0 1 1 0],[0 0 1 1],c1);patch([0 1 1 1-e 1-e 0+e],[0 0 1 1-e 0+e 0+e],c2);patch([0 0 1 1-e 0+e 0+e],[0 1 1 1-e 1-e 0+e],c3);plot([0 1 1 0 0],[0 0 1 1 0]);disp('weights');
  "IW{1,1}(5,:)'" : Constant  Value=[-0.0167471374249104666687149034487447352148592472076416015625;-0.1403490032915202523344788687609252519905567169189453125;0.06539080578002652577307429737629718147218227386474609375;-0.1072757424021300864946937281274585984647274017333984375;-0.187929354284938898711487809123354963958263397216796875;-0.381491903135239507349751875153742730617523193359375;0.049629414578369744626140658283475204370915889739990234375;-0.41530209335088208444375368344481103122234344482421875;-0.23323378805868311136606507716351188719272613525390625;0.05655189496379055269503766112393350340425968170166015625;-0.0308493821346236575531296608687625848688185214996337890625;0.394529092626329236370708031245158053934574127197265625;-0.49345783741323645532617092612781561911106109619140625;-0.1584317625033743459628254868221119977533817291259765625;0.0061863610017271232488500487534111016429960727691650390625;0.45637564416267084599354575402685441076755523681640625;-0.50470661977217912141924216484767384827136993408203125;0.5152242785644964850888527507777325809001922607421875;0.445594108186020132489346678994479589164257049560546875;-0.39961123621634764280230456279241479933261871337890625]
      mask Display: e = 0.06;c1 = [120 150 230]/255;c2 = ([120 150 230]+0)/383;c3 = ([120 150 230]+128)/383;patch([0 1 1 0],[0 0 1 1],c1);patch([0 1 1 1-e 1-e 0+e],[0 0 1 1-e 0+e 0+e],c2);patch([0 0 1 1-e 0+e 0+e],[0 1 1 1-e 1-e 0+e],c3);plot([0 1 1 0 0],[0 0 1 1 0]);disp('weights');
  "IW{1,1}(6,:)'" : Constant  Value=[0.3981536228839750446439893494243733584880828857421875;-0.463262998085407551318581909072236157953739166259765625;0.307467747633039134580457130141439847648143768310546875;0.19670090243097793081261670522508211433887481689453125;-0.07431367785636679157423856167952180840075016021728515625;-0.30532129558632081778313249742495827376842498779296875;-0.32232627374899125438645342001109384000301361083984375;0.2971313393515180312220991254434920847415924072265625;-0.2392597967351715038120119061204604804515838623046875;-0.419141866007090302392867897651740349829196929931640625;0.322875854212182067382030936641967855393886566162109375;-0.1904395935907823023125473582695121876895427703857421875;-0.1818347259374590851876973829348571598529815673828125;0.415873410567199897069912140068481676280498504638671875;0.322350419715700386991130699243512935936450958251953125;0.2081847913596024113314086889658938162028789520263671875;-0.446763843250777947790908228853368200361728668212890625;-0.33915665318155541196887270416482351720333099365234375;0.121639126546729148259373687324114143848419189453125;0.1740472985364560909449238579327357001602649688720703125]
      mask Display: e = 0.06;c1 = [120 150 230]/255;c2 = ([120 150 230]+0)/383;c3 = ([120 150 230]+128)/383;patch([0 1 1 0],[0 0 1 1],c1);patch([0 1 1 1-e 1-e 0+e],[0 0 1 1-e 0+e 0+e],c2);patch([0 0 1 1-e 0+e 0+e],[0 1 1 1-e 1-e 0+e],c3);plot([0 1 1 0 0],[0 0 1 1 0]);disp('weights');
  "IW{1,1}(7,:)'" : Constant  Value=[0.376732950367336727470757296032388694584369659423828125;-0.34110606780804475501867045750259421765804290771484375;-0.428897245916350533523342392072663642466068267822265625;-0.42202281742953717813549019410856999456882476806640625;0.09229029021692945755628301185424788855016231536865234375;-0.28676061684988851663291598015348426997661590576171875;-0.258405950729481137528864564956165850162506103515625;0.399879661150548237902313530867104418575763702392578125;0.35239904278103229007257368721184320747852325439453125;-0.438546522706632024846129525030846707522869110107421875;-0.390045347549494214600684927063412033021450042724609375;-0.0981691829835769080858653978793881833553314208984375;0.394358315572709450247401719025219790637493133544921875;-0.248659614140606610721562219623592682182788848876953125;0.34202493685243073873181174349156208336353302001953125;-0.32053968374792785045457321757567115128040313720703125;0.25316722915738998356260935906902886927127838134765625;0.41502683282907881778811542972107417881488800048828125;-0.07079259195542830784830812262953259050846099853515625;0.2492476841982780022544119447047705762088298797607421875]
      mask Display: e = 0.06;c1 = [120 150 230]/255;c2 = ([120 150 230]+0)/383;c3 = ([120 150 230]+128)/383;patch([0 1 1 0],[0 0 1 1],c1);patch([0 1 1 1-e 1-e 0+e],[0 0 1 1-e 0+e 0+e],c2);patch([0 0 1 1-e 0+e 0+e],[0 1 1 1-e 1-e 0+e],c3);plot([0 1 1 0 0],[0 0 1 1 0]);disp('weights');
  "IW{1,1}(8,:)'" : Constant  Value=[0.03936558636368105157377073055613436736166477203369140625;0.377442071789987065866256443769088946282863616943359375;0.284083965870056298630430546836578287184238433837890625;0.581018667978522973527333306265063583850860595703125;-0.50854269744919256002191332299844361841678619384765625;0.32517991331879481098354744972311891615390777587890625;0.07405993707905016154580124521089601330459117889404296875;0.556143558134105209234121502959169447422027587890625;-0.003167755148407028382984140790767924045212566852569580078125;-0.5360407465765650858458002403494901955127716064453125;-0.0972922773624158299110575853774207644164562225341796875;-0.299269339530805922322542755864560604095458984375;0.25071749302060786224188859705463983118534088134765625;0.465564615412748905587392300731153227388858795166015625;-0.261402281606591013751739183135214261710643768310546875;0.345097368461358355862245161915780045092105865478515625;0.1767640433081788808866718909484916366636753082275390625;0.04380173619142592456032758718720288015902042388916015625;-0.1410128778417972517100764662245637737214565277099609375;0.0310970269928661779967882239361642859876155853271484375]
      mask Display: e = 0.06;c1 = [120 150 230]/255;c2 = ([120 150 230]+0)/383;c3 = ([120 150 230]+128)/383;patch([0 1 1 0],[0 0 1 1],c1);patch([0 1 1 1-e 1-e 0+e],[0 0 1 1-e 0+e 0+e],c2);patch([0 0 1 1-e 0+e 0+e],[0 1 1 1-e 1-e 0+e],c3);plot([0 1 1 0 0],[0 0 1 1 0]);disp('weights');
  "IW{1,1}(9,:)'" : Constant  Value=[0.4824204354555963192296985653229057788848876953125;-0.03494619306651880474845484059187583625316619873046875;-0.2174074457393145587413840758017613552510738372802734375;-0.210770258029754631312613355476059950888156890869140625;0.350617376357728105507050031519611366093158721923828125;-0.1497310545967961703528459338485845364630222320556640625;0.287690321438704488254956004311679862439632415771484375;0.0647101088775734745173195960887824185192584991455078125;-0.10804537864294576354762256187314051203429698944091796875;-0.48185501228065874546047098192502744495868682861328125;-0.433809439795235174397447508454206399619579315185546875;-0.0283275030564603437499560101286988356150686740875244140625;0.489137501633702453940344412330887280404567718505859375;0.395445520839683928304708615542040206491947174072265625;0.4073316471249626147255185060203075408935546875;0.281986325445919561172303247076342813670635223388671875;-0.352615414049573139276816391429747454822063446044921875;0.4117400328493265870832829023129306733608245849609375;0.463338716754537915942790959888952784240245819091796875;-0.328692084280040541788281416302197612822055816650390625]
      mask Display: e = 0.06;c1 = [120 150 230]/255;c2 = ([120 150 230]+0)/383;c3 = ([120 150 230]+128)/383;patch([0 1 1 0],[0 0 1 1],c1);patch([0 1 1 1-e 1-e 0+e],[0 0 1 1-e 0+e 0+e],c2);patch([0 0 1 1-e 0+e 0+e],[0 1 1 1-e 1-e 0+e],c3);plot([0 1 1 0 0],[0 0 1 1 0]);disp('weights');
  Mux : Mux  Inputs=20
      mask Display: e = 0.06;c1 = [120 150 230]/255;c2 = ([120 150 230]+0)/383;c3 = ([120 150 230]+128)/383;patch([0 1 1 0],[0 0 1 1],c1);patch([0 1 1 1-e 1-e 0+e],[0 0 1 1-e 0+e 0+e],c2);patch([0 0 1 1-e 0+e 0+e],[0 1 1 1-e 1-e 0+e],c3);plot([0 1 1 0 0],[0 0 1 1 0]);disp('Mux');
  dotprod{1..20} (20 alike) : neural/Weight Functions/dotprod
  "lz{1,1}" : Outport
      mask Display: e = 0.06;c1 = [120 230 180]/255;c2 = ([120 230 180]+0)/(256+128);c3 = ([120 230 180]+128)/(256+128);patch([0 1 1 0],[0 0 1 1],c1);patch([0 1 1 1-e 1-e 0+e],[0 0 1 1-e 0+e 0+e],c2);patch([0 0 1 1-e 0+e 0+e],[0 1 1 1-e 1-e 0+e],c3);plot([0 1 1 0 0],[0 0 1 1 0]);
  wires:
  "IW{1,1}(1,:)'"/1 -> dotprod1/1
  "ad{1,1}"/1 -> dotprod1/2, dotprod2/2, dotprod3/2, dotprod4/2, dotprod5/2, dotprod6/2, dotprod7/2, dotprod8/2, dotprod9/2, dotprod10/2, dotprod11/2, dotprod12/2, dotprod13/2, dotprod14/2, dotprod15/2, dotprod16/2, dotprod17/2, dotprod18/2, dotprod19/2, dotprod20/2
  dotprod1/1 -> Mux/1
  "IW{1,1}(2,:)'"/1 -> dotprod2/1
  dotprod2/1 -> Mux/2
  "IW{1,1}(3,:)'"/1 -> dotprod3/1
  dotprod3/1 -> Mux/3
  "IW{1,1}(4,:)'"/1 -> dotprod4/1
  dotprod4/1 -> Mux/4
  "IW{1,1}(5,:)'"/1 -> dotprod5/1
  dotprod5/1 -> Mux/5
  "IW{1,1}(6,:)'"/1 -> dotprod6/1
  dotprod6/1 -> Mux/6
  "IW{1,1}(7,:)'"/1 -> dotprod7/1
  dotprod7/1 -> Mux/7
  "IW{1,1}(8,:)'"/1 -> dotprod8/1
  dotprod8/1 -> Mux/8
  "IW{1,1}(9,:)'"/1 -> dotprod9/1
  dotprod9/1 -> Mux/9
  "IW{1,1}(10,:)'"/1 -> dotprod10/1
  dotprod10/1 -> Mux/10
  "IW{1,1}(11,:)'"/1 -> dotprod11/1
  dotprod11/1 -> Mux/11
  "IW{1,1}(12,:)'"/1 -> dotprod12/1
  dotprod12/1 -> Mux/12
  "IW{1,1}(13,:)'"/1 -> dotprod13/1
  dotprod13/1 -> Mux/13
  "IW{1,1}(14,:)'"/1 -> dotprod14/1
  dotprod14/1 -> Mux/14
  "IW{1,1}(15,:)'"/1 -> dotprod15/1
  dotprod15/1 -> Mux/15
  "IW{1,1}(16,:)'"/1 -> dotprod16/1
  dotprod16/1 -> Mux/16
  "IW{1,1}(17,:)'"/1 -> dotprod17/1
  dotprod17/1 -> Mux/17
  "IW{1,1}(18,:)'"/1 -> dotprod18/1
  dotprod18/1 -> Mux/18
  "IW{1,1}(19,:)'"/1 -> dotprod19/1
  dotprod19/1 -> Mux/19
  "IW{1,1}(20,:)'"/1 -> dotprod20/1
  dotprod20/1 -> Mux/20
  Mux/1 -> "lz{1,1}"/1

== system Copy_of_compare/Subsystem2/Custom Neural Network/Layer 2/Delays 1 ==
  "p{2}" : Inport  PortDimensions=20  SampleTime=1
      mask Display: e = 0.06;c1 = [120 230 180]/255;c2 = ([120 230 180]+0)/(256+128);c3 = ([120 230 180]+128)/(256+128);patch([0 1 1 0],[0 0 1 1],c1);patch([0 1 1 1-e 1-e 0+e],[0 0 1 1-e 0+e 0+e],c2);patch([0 0 1 1-e 0+e 0+e],[0 1 1 1-e 1-e 0+e],c3);plot([0 1 1 0 0],[0 0 1 1 0]);
  mux : Mux  Inputs=1
      mask Display: e = 0.06;c1 = [120 150 230]/255;c2 = ([120 150 230]+0)/383;c3 = ([120 150 230]+128)/383;patch([0 1 1 0],[0 0 1 1],c1);patch([0 1 1 1-e 1-e 0+e],[0 0 1 1-e 0+e 0+e],c2);patch([0 0 1 1-e 0+e 0+e],[0 1 1 1-e 1-e 0+e],c3);plot([0 1 1 0 0],[0 0 1 1 0]);disp('Mux')
  "pd{2,1}" : Outport
      mask Display: e = 0.06;c1 = [120 230 180]/255;c2 = ([120 230 180]+0)/(256+128);c3 = ([120 230 180]+128)/(256+128);patch([0 1 1 0],[0 0 1 1],c1);patch([0 1 1 1-e 1-e 0+e],[0 0 1 1-e 0+e 0+e],c2);patch([0 0 1 1-e 0+e 0+e],[0 1 1 1-e 1-e 0+e],c3);plot([0 1 1 0 0],[0 0 1 1 0]);
  wires:
  "p{2}"/1 -> mux/1
  mux/1 -> "pd{2,1}"/1

== system Copy_of_compare/Subsystem2/Custom Neural Network/Layer 2/Delays 2 ==
  "p{2}" : Inport  PortDimensions=15  SampleTime=1
      mask Display: e = 0.06;c1 = [120 230 180]/255;c2 = ([120 230 180]+0)/(256+128);c3 = ([120 230 180]+128)/(256+128);patch([0 1 1 0],[0 0 1 1],c1);patch([0 1 1 1-e 1-e 0+e],[0 0 1 1-e 0+e 0+e],c2);patch([0 0 1 1-e 0+e 0+e],[0 1 1 1-e 1-e 0+e],c3);plot([0 1 1 0 0],[0 0 1 1 0]);
  Delay 1 : UnitDelay  InitialCondition=ai_layer_2_delayed_1
      mask Display: e = 0.06;c1 = [120 150 230]/255;c2 = ([120 150 230]+0)/383;c3 = ([120 150 230]+128)/383;patch([0 1 1 0],[0 0 1 1],c1);patch([0 1 1 1-e 1-e 0+e],[0 0 1 1-e 0+e 0+e],c2);patch([0 0 1 1-e 0+e 0+e],[0 1 1 1-e 1-e 0+e],c3);plot([0 1 1 0 0],[0 0 1 1 0]);disp('D')
  mux : Mux  Inputs=1
      mask Display: e = 0.06;c1 = [120 150 230]/255;c2 = ([120 150 230]+0)/383;c3 = ([120 150 230]+128)/383;patch([0 1 1 0],[0 0 1 1],c1);patch([0 1 1 1-e 1-e 0+e],[0 0 1 1-e 0+e 0+e],c2);patch([0 0 1 1-e 0+e 0+e],[0 1 1 1-e 1-e 0+e],c3);plot([0 1 1 0 0],[0 0 1 1 0]);disp('Mux')
  "pd{2,2}" : Outport
      mask Display: e = 0.06;c1 = [120 230 180]/255;c2 = ([120 230 180]+0)/(256+128);c3 = ([120 230 180]+128)/(256+128);patch([0 1 1 0],[0 0 1 1],c1);patch([0 1 1 1-e 1-e 0+e],[0 0 1 1-e 0+e 0+e],c2);patch([0 0 1 1-e 0+e 0+e],[0 1 1 1-e 1-e 0+e],c3);plot([0 1 1 0 0],[0 0 1 1 0]);
  wires:
  "p{2}"/1 -> Delay 1/1
  Delay 1/1 -> mux/1
  mux/1 -> "pd{2,2}"/1
